simulink model "ProgrammentwurfMatlab"  (R2025b)
settings: Solver=VariableStepAuto  StartTime=0.0  StopTime=3  RelTol=1e-8
libraries: simulink x2
settings Model: Creator=jonas  LastModifiedBy=fisch

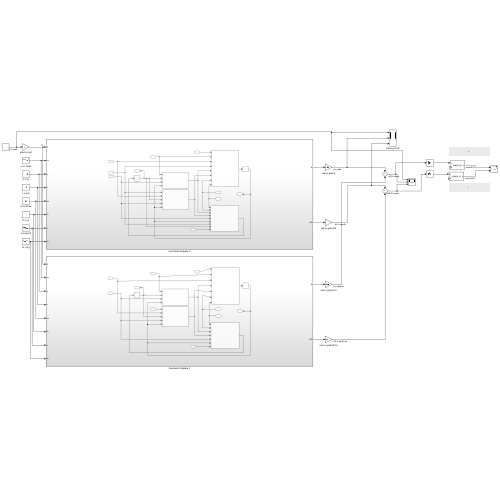
[thumbnail: Simulink's stored preview of the top-level diagram]
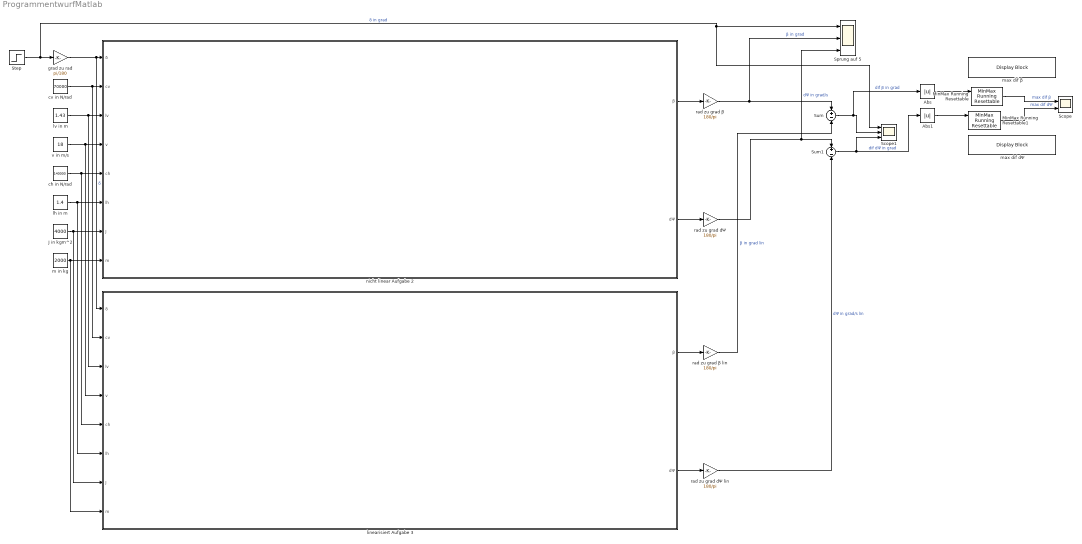
== system ProgrammentwurfMatlab ==
  Abs : Abs  SaturateOnIntegerOverflow=off
  Abs1 : Abs  SaturateOnIntegerOverflow=off
  J in kgm^2 : Constant  Value=4000
  MinMax Running Resettable : simulink/Math Operations/MinMax Running Resettable  Function=max  vinit=0.0
  MinMax Running Resettable1 : simulink/Math Operations/MinMax Running Resettable  Function=max  vinit=0.0
  Scope : Scope  NumInputPorts=2
      settings: ActiveDisplayYMinimum=-0.45477  ActiveDisplayYMaximum=4.09297  DataLoggingVariableName=ScopeData2
  Scope1 : Scope  NumInputPorts=3
      settings: ActiveDisplayYMinimum=-6.59297  ActiveDisplayYMaximum=22.95477
  Sprung auf 5 : Scope  NumInputPorts=3
      settings: ActiveDisplayYMinimum=-12.49053  ActiveDisplayYMaximum=78.26951
  Step : Step  SampleTime=0
  Sum : Sum  Inputs=+|-
  Sum1 : Sum  Inputs=+|-
  ch in N/rad : Constant  Value=140000
  cv in N/rad : Constant  Value=70000
  grad zu rad : Gain  Gain=pi/180
  lh in m : Constant  Value=1.4
  linearisiert Aufgabe 3 : Subsystem
  lv in m : Constant  Value=1.43
  m in kg : Constant  Value=2000
  max dif dΨ : DisplayBlock  LabelPosition=Hide  Transparency=1  GridColor=[0.502, 0.502, 0.502]
  max dif β : DisplayBlock  LabelPosition=Hide  Transparency=1  GridColor=[0.502, 0.502, 0.502]
  nicht linear Aufgabe 2 : Subsystem
  rad zu grad dΨ : Gain  Gain=180/pi
  rad zu grad dΨ lin : Gain  Gain=180/pi
  rad zu grad β : Gain  Gain=180/pi
  rad zu grad β lin : Gain  Gain=180/pi
  v in m/s : Constant  Value=18
  wires:
  Step/1 -> Scope1/1, Sprung auf 5/1, grad zu rad/1  "δ in grad"
  rad zu grad β/1 -> Sprung auf 5/2, Sum/1  "β in grad"
  rad zu grad dΨ/1 -> Sprung auf 5/3, Sum1/1  "dΨ in grad/s"
  grad zu rad/1 -> linearisiert Aufgabe 3/1(δ), nicht linear Aufgabe 2/1(δ)  "δ"
  cv in N/rad/1 -> linearisiert Aufgabe 3/2(cv), nicht linear Aufgabe 2/2(cv)
  lv in m/1 -> linearisiert Aufgabe 3/3(lv), nicht linear Aufgabe 2/3(lv)
  v in m/s/1 -> linearisiert Aufgabe 3/4(v), nicht linear Aufgabe 2/4(v)
  ch in N/rad/1 -> linearisiert Aufgabe 3/5(ch), nicht linear Aufgabe 2/5(ch)
  lh in m/1 -> linearisiert Aufgabe 3/6(lh), nicht linear Aufgabe 2/6(lh)
  J in kgm^2/1 -> linearisiert Aufgabe 3/7(J), nicht linear Aufgabe 2/7(J)
  m in kg/1 -> linearisiert Aufgabe 3/8(m), nicht linear Aufgabe 2/8(m)
  nicht linear Aufgabe 2/1(β) -> rad zu grad β/1
  nicht linear Aufgabe 2/2(dΨ) -> rad zu grad dΨ/1
  linearisiert Aufgabe 3/1(β) -> rad zu grad β lin/1
  linearisiert Aufgabe 3/2(dΨ) -> rad zu grad dΨ lin/1
  rad zu grad β lin/1 -> Sum/2  "β in grad lin"
  rad zu grad dΨ lin/1 -> Sum1/2  "dΨ in grad/s lin"
  Sum1/1 -> Abs1/1, Scope1/3  "dif dΨ in grad"
  Sum/1 -> Abs/1, Scope1/2  "dif β in grad"
  Abs/1 -> MinMax Running Resettable/1
  Abs1/1 -> MinMax Running Resettable1/1
  MinMax Running Resettable/1 -> Scope/1  "max dif β"
  MinMax Running Resettable1/1 -> Scope/2  "max dif dΨ"

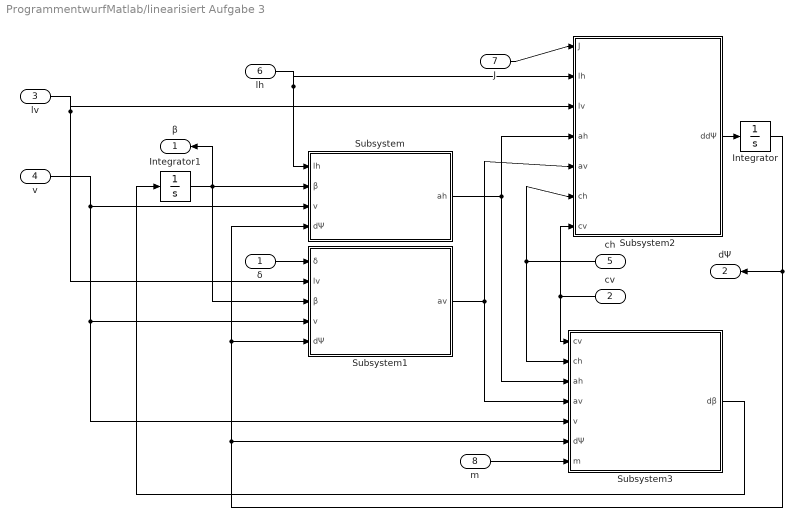
== system ProgrammentwurfMatlab/linearisiert Aufgabe 3 ==
  δ : Inport
  cv : Inport  Port=2
  lv : Inport  Port=3
  v : Inport  Port=4
  ch : Inport  Port=5
  lh : Inport  Port=6
  J : Inport  Port=7
  m : Inport  Port=8
  Integrator : Integrator
  Integrator1 : Integrator
  Subsystem : Subsystem
  Subsystem1 : Subsystem
  Subsystem2 : Subsystem
  Subsystem3 : Subsystem
  β : Outport
  dΨ : Outport  Port=2
  wires:
  Subsystem3/1(dβ) -> Integrator1/1
  Subsystem/1(ah) -> Subsystem3/3(ah), Subsystem2/4(ah)
  ch/1 -> Subsystem2/6(ch), Subsystem3/2(ch)
  Integrator/1 -> Subsystem3/6(dΨ), Subsystem1/5(dΨ), Subsystem/4(dΨ), dΨ/1
  Subsystem2/1(ddΨ) -> Integrator/1
  Integrator1/1 -> Subsystem/2(β), Subsystem1/3(β), β/1
  δ/1 -> Subsystem1/1(δ)
  lh/1 -> Subsystem/1(lh), Subsystem2/2(lh)
  Subsystem1/1(av) -> Subsystem3/4(av), Subsystem2/5(av)
  lv/1 -> Subsystem1/2(lv), Subsystem2/3(lv)
  cv/1 -> Subsystem2/7(cv), Subsystem3/1(cv)
  J/1 -> Subsystem2/1(J)
  v/1 -> Subsystem3/5(v), Subsystem1/4(v), Subsystem/3(v)
  m/1 -> Subsystem3/7(m)

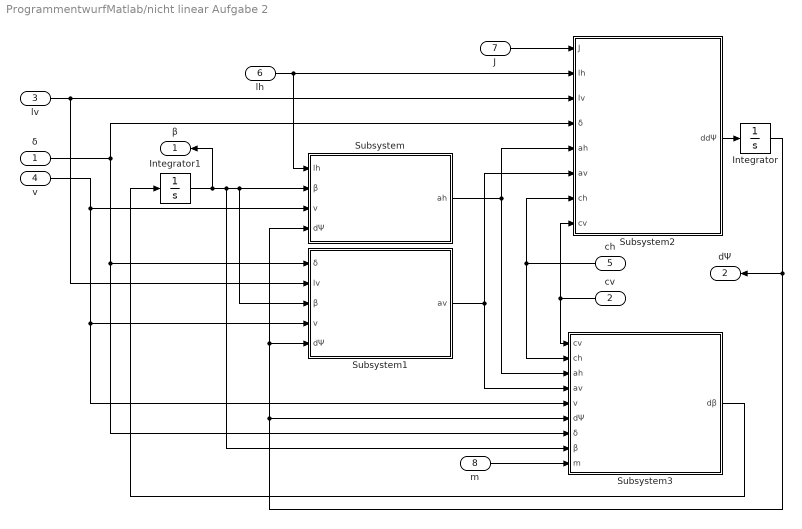
== system ProgrammentwurfMatlab/nicht linear Aufgabe 2 ==
  δ : Inport
  cv : Inport  Port=2
  lv : Inport  Port=3
  v : Inport  Port=4
  ch : Inport  Port=5
  lh : Inport  Port=6
  J : Inport  Port=7
  m : Inport  Port=8
  Integrator : Integrator
  Integrator1 : Integrator
  Subsystem : Subsystem
  Subsystem1 : Subsystem
  Subsystem2 : Subsystem
  Subsystem3 : Subsystem
  β : Outport
  dΨ : Outport  Port=2
  wires:
  Subsystem3/1(dβ) -> Integrator1/1
  Subsystem/1(ah) -> Subsystem3/3(ah), Subsystem2/5(ah)
  ch/1 -> Subsystem2/7(ch), Subsystem3/2(ch)
  Integrator/1 -> Subsystem/4(dΨ), Subsystem1/5(dΨ), Subsystem3/6(dΨ), dΨ/1
  Subsystem2/1(ddΨ) -> Integrator/1
  Integrator1/1 -> Subsystem3/8(β), Subsystem/2(β), Subsystem1/3(β), β/1
  δ/1 -> Subsystem2/4(δ), Subsystem3/7(δ), Subsystem1/1(δ)
  lh/1 -> Subsystem/1(lh), Subsystem2/2(lh)
  Subsystem1/1(av) -> Subsystem3/4(av), Subsystem2/6(av)
  lv/1 -> Subsystem1/2(lv), Subsystem2/3(lv)
  cv/1 -> Subsystem2/8(cv), Subsystem3/1(cv)
  J/1 -> Subsystem2/1(J)
  v/1 -> Subsystem3/5(v), Subsystem1/4(v), Subsystem/3(v)
  m/1 -> Subsystem3/9(m)

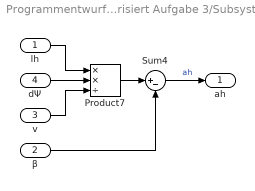
== system ProgrammentwurfMatlab/linearisiert Aufgabe 3/Subsystem ==
  lh : Inport
  β : Inport  Port=2
  v : Inport  Port=3
  dΨ : Inport  Port=4
  Product7 : Product  Inputs=**/
  Sum4 : Sum  Inputs=|+-
  ah : Outport
  wires:
  Product7/1 -> Sum4/1
  dΨ/1 -> Product7/2
  β/1 -> Sum4/2
  lh/1 -> Product7/1
  v/1 -> Product7/3
  Sum4/1 -> ah/1  "ah"

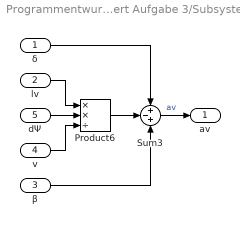
== system ProgrammentwurfMatlab/linearisiert Aufgabe 3/Subsystem1 ==
  δ : Inport
  lv : Inport  Port=2
  β : Inport  Port=3
  v : Inport  Port=4
  dΨ : Inport  Port=5
  Product6 : Product  Inputs=**/
  Sum3 : Sum  Inputs=+-+
  av : Outport
  wires:
  lv/1 -> Product6/1
  β/1 -> Sum3/3
  Product6/1 -> Sum3/2
  dΨ/1 -> Product6/2
  Sum3/1 -> av/1  "av"
  v/1 -> Product6/3
  δ/1 -> Sum3/1

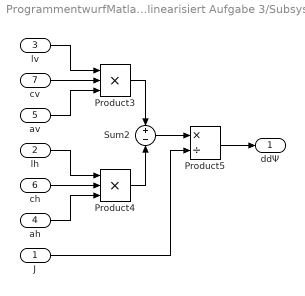
== system ProgrammentwurfMatlab/linearisiert Aufgabe 3/Subsystem2 ==
  J : Inport
  lh : Inport  Port=2
  lv : Inport  Port=3
  ah : Inport  Port=4
  av : Inport  Port=5
  ch : Inport  Port=6
  cv : Inport  Port=7
  Product3 : Product  Inputs=***
  Product4 : Product  Inputs=***
  Product5 : Product  Inputs=*/
  Sum2 : Sum  Inputs=+|-
  ddΨ : Outport
  wires:
  Sum2/1 -> Product5/1
  av/1 -> Product3/3
  ch/1 -> Product4/2
  lh/1 -> Product4/1
  Product3/1 -> Sum2/1
  cv/1 -> Product3/2
  Product4/1 -> Sum2/2
  ah/1 -> Product4/3
  Product5/1 -> ddΨ/1
  lv/1 -> Product3/1
  J/1 -> Product5/2

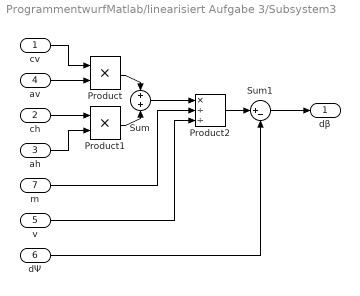
== system ProgrammentwurfMatlab/linearisiert Aufgabe 3/Subsystem3 ==
  cv : Inport
  ch : Inport  Port=2
  ah : Inport  Port=3
  av : Inport  Port=4
  v : Inport  Port=5
  dΨ : Inport  Port=6
  m : Inport  Port=7
  Product : Product  Inputs=**
  Product1 : Product  Inputs=**
  Product2 : Product  Inputs=*//
  Sum : Sum  Inputs=+|+
  Sum1 : Sum  Inputs=|+-
  dβ : Outport
  wires:
  Product/1 -> Sum/1
  m/1 -> Product2/2
  cv/1 -> Product/1
  Product2/1 -> Sum1/1
  Product1/1 -> Sum/2
  Sum/1 -> Product2/1
  Sum1/1 -> dβ/1
  av/1 -> Product/2
  v/1 -> Product2/3
  dΨ/1 -> Sum1/2
  ah/1 -> Product1/2
  ch/1 -> Product1/1

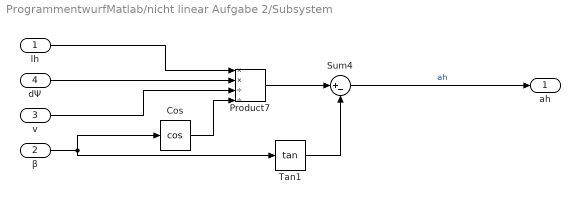
== system ProgrammentwurfMatlab/nicht linear Aufgabe 2/Subsystem ==
  lh : Inport
  β : Inport  Port=2
  v : Inport  Port=3
  dΨ : Inport  Port=4
  Cos : Trigonometry  Operator=cos
  Product7 : Product  Inputs=**//
  Sum4 : Sum  Inputs=|+-
  Tan1 : Trigonometry  Operator=tan
  ah : Outport
  wires:
  Cos/1 -> Product7/4
  Product7/1 -> Sum4/1
  dΨ/1 -> Product7/2
  Tan1/1 -> Sum4/2
  lh/1 -> Product7/1
  v/1 -> Product7/3
  Sum4/1 -> ah/1  "ah"
  β/1 -> Tan1/1, Cos/1

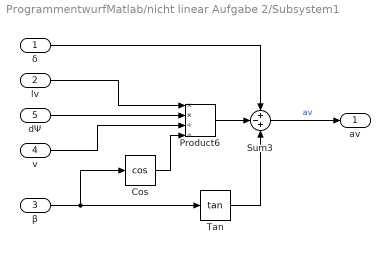
== system ProgrammentwurfMatlab/nicht linear Aufgabe 2/Subsystem1 ==
  δ : Inport
  lv : Inport  Port=2
  β : Inport  Port=3
  v : Inport  Port=4
  dΨ : Inport  Port=5
  Cos : Trigonometry  Operator=cos
  Product6 : Product  Inputs=**//
  Sum3 : Sum  Inputs=+-+
  Tan : Trigonometry  Operator=tan
  av : Outport
  wires:
  lv/1 -> Product6/1
  Tan/1 -> Sum3/3
  Product6/1 -> Sum3/2
  dΨ/1 -> Product6/2
  Sum3/1 -> av/1  "av"
  v/1 -> Product6/3
  β/1 -> Cos/1, Tan/1
  δ/1 -> Sum3/1
  Cos/1 -> Product6/4

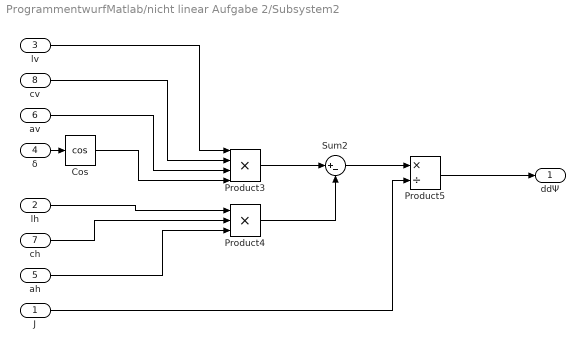
== system ProgrammentwurfMatlab/nicht linear Aufgabe 2/Subsystem2 ==
  J : Inport
  lh : Inport  Port=2
  lv : Inport  Port=3
  δ : Inport  Port=4
  ah : Inport  Port=5
  av : Inport  Port=6
  ch : Inport  Port=7
  cv : Inport  Port=8
  Cos : Trigonometry  Operator=cos
  Product3 : Product  Inputs=****
  Product4 : Product  Inputs=***
  Product5 : Product  Inputs=*/
  Sum2 : Sum  Inputs=|+-
  ddΨ : Outport
  wires:
  Sum2/1 -> Product5/1
  av/1 -> Product3/3
  ch/1 -> Product4/2
  lh/1 -> Product4/1
  Product3/1 -> Sum2/1
  cv/1 -> Product3/2
  Product4/1 -> Sum2/2
  ah/1 -> Product4/3
  Product5/1 -> ddΨ/1
  lv/1 -> Product3/1
  J/1 -> Product5/2
  δ/1 -> Cos/1
  Cos/1 -> Product3/4

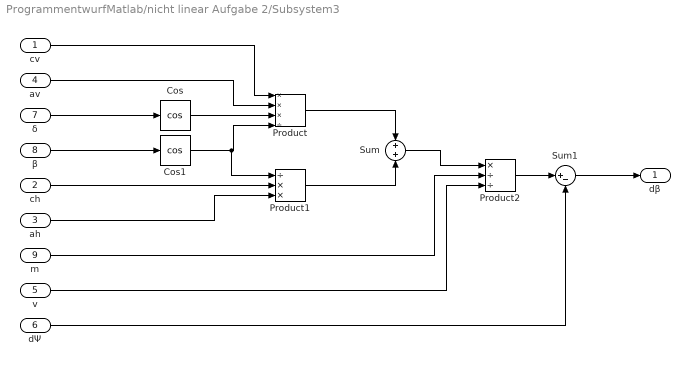
== system ProgrammentwurfMatlab/nicht linear Aufgabe 2/Subsystem3 ==
  cv : Inport
  ch : Inport  Port=2
  ah : Inport  Port=3
  av : Inport  Port=4
  v : Inport  Port=5
  dΨ : Inport  Port=6
  δ : Inport  Port=7
  β : Inport  Port=8
  m : Inport  Port=9
  Cos : Trigonometry  Operator=cos
  Cos1 : Trigonometry  Operator=cos
  Product : Product  Inputs=***/
  Product1 : Product  Inputs=/**
  Product2 : Product  Inputs=*//
  Sum : Sum  Inputs=+|+
  Sum1 : Sum  Inputs=|+-
  dβ : Outport
  wires:
  Product/1 -> Sum/1
  m/1 -> Product2/2
  cv/1 -> Product/1
  Product2/1 -> Sum1/1
  Product1/1 -> Sum/2
  Sum/1 -> Product2/1
  Sum1/1 -> dβ/1
  av/1 -> Product/2
  v/1 -> Product2/3
  dΨ/1 -> Sum1/2
  δ/1 -> Cos/1
  β/1 -> Cos1/1
  Cos/1 -> Product/3
  Cos1/1 -> Product1/1, Product/4
  ch/1 -> Product1/2
  ah/1 -> Product1/3
